simulink subsystem "PMSM"  (R2023b)
settings: Solver=VariableStepAuto  StartTime=0.0  StopTime=10.0  RelTol=1e-3
libraries: spsPermanentMagnetSynchronousMachineLib x1
settings Model: Creator=rainy  LastModifiedBy=rainy

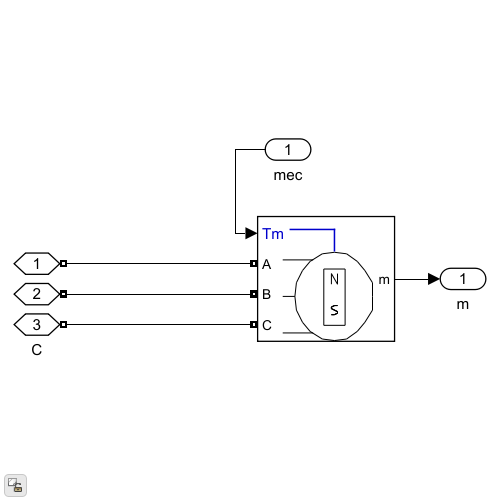
[thumbnail: Simulink's stored preview of the top-level diagram]
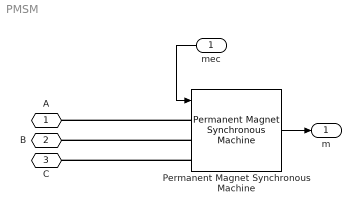
== system PMSM ==
  mec : Inport
  Permanent Magnet Synchronous Machine : spsPermanentMagnetSynchronousMachineLib/Permanent Magnet Synchronous Machine  NbPhases=3  FluxDistribution=Sinusoidal  RotorType=Round  MechanicalLoad=Torque Tm  PresetModel=No  ShowDetailedParameters=on  MeasurementBus=off  Resistance=1.2  Inductance=8.5e-3  dqInductances=[8.5e-3,8.5e-3]  La=8.5e-3  MachineConstant=Flux linkage established by magnets (V.s)  Flux=0.175  VoltageCst=126.966  TorqueCst=1.05  Flat=120  Mechanical=[0.0008 0.0004924 4 0]  PolePairs=4  InitialConditions=[0,0, 0,0]  InitialConditions5ph=[0 0 0 0 0 0]  RefAngle=Aligned with phase A axis (original Park)  IterativeDiscreteModel=Trapezoidal non iterative  TsBlock=-1  TsPowergui=0
  A : PMIOPort  Side=Left
  B : PMIOPort  Port=2  Side=Left
  C : PMIOPort  Port=3  Side=Left
  m : Outport
  wires:
  Permanent Magnet Synchronous Machine/1 -> m/1
  mec/1 -> Permanent Magnet Synchronous Machine/1
  connections:
  Permanent Magnet Synchronous Machine/LConn2 -- B/RConn1
  Permanent Magnet Synchronous Machine/LConn1 -- A/RConn1
  Permanent Magnet Synchronous Machine/LConn3 -- C/RConn1
